simulink model "vab_to_uvw_test"  (R2017a)
settings: Solver=VariableStepAuto  StartTime=0.0  StopTime=10.0  RelTol=1e-3
settings Model: Creator=mudat  LastModifiedBy=mudat

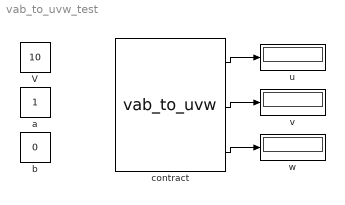
== system vab_to_uvw_test ==
  V : Constant  Value=10
  a : Constant
  b : Constant  Value=0
  contract : M-S-Function  FunctionName=vab_to_uvw  mask{assumePorts=4}
      mask prompts: assumePorts "Assume ports"
      mask Callback assumePorts: contract_callback('assume_callback',gcb)
      mask Display:
      | port_label('input',1,'assume')
      | port_label('input',2,'assume')
      | port_label('input',3,'assume')
      | port_label('input',4,'assume')
  u : Display
  v : Display
  w : Display
  wires:
  contract/1 -> u/1
  contract/2 -> v/1
  contract/3 -> w/1
